simulink model "TRAMI_TM_PNT"  (R2018b)
settings: Solver=ode8  StartTime=0  StopTime=end_time  FixedStep=sampling_time  RelTol=1e-3
PreLoadFcn:
  | TRAMI_TM_PNT_PreLoad;
values from neighbouring files (symbols this model uses):
  sampling_time = 0.0025    [METI_TRAMI_Thermal_ver01_Jmaab_PreLoad.m]
settings Model: Creator=nishimura  LastModifiedBy=E00026
settings DataIOCC: LimitDataPoints=on  SaveFormat=Array  SaveOutput=off  InspectSignalLogs=on  SaveTime=off
settings OptimizationCC: BlockReduction=off  BooleanDataType=off  LifeSpan=inf
settings DebuggingCC: SaveWithParameterizedLinksMsg=none  UnderspecifiedInitializationDetection=Classic  MergeDetectMultiDrivingBlocksExec=none  SignalResolutionControl=TryResolveAllWithWarning  ParameterPrecisionLossMsg=none  StrictBusMsg=ErrorOnBusTreatedAsVector  SFUnexpectedBacktrackingDiag=warning  SFNoUnconditionalDefaultTransitionDiag=warning  SFExecutionAtInitializationDiag=none
settings HardwareCC: ProdBitPerPointer=32  ProdBitPerSizeT=32  ProdBitPerPtrDiffT=32  ProdLargestAtomicFloat=None  ProdIntDivRoundTo=Undefined  ProdEndianess=Unspecified  ProdWordSize=32  ProdHWDeviceType=32-bit Generic  TargetUnknown=on
settings ModelReferenceCC: PropagateSignalLabelsOutOfModel=off
settings SFSimCC: SimUseLocalCustomCode=off
settings RTWCC: RTWUseLocalCustomCode=off
settings CodeAppCC: StateflowObjectComments=on
settings GRTTargetCC: TargetLangStandard=C89/C90 (ANSI)  GeneratePreprocessorConditionals=Disable all
settings ConfigComp: CovMetricSettings=dw  CovHtmlReporting=on  CovSaveCumulativeToWorkspaceVar=on  CovSaveSingleToWorkspaceVar=on  CovExternalEMLEnable=off  CovSFcnEnable=off

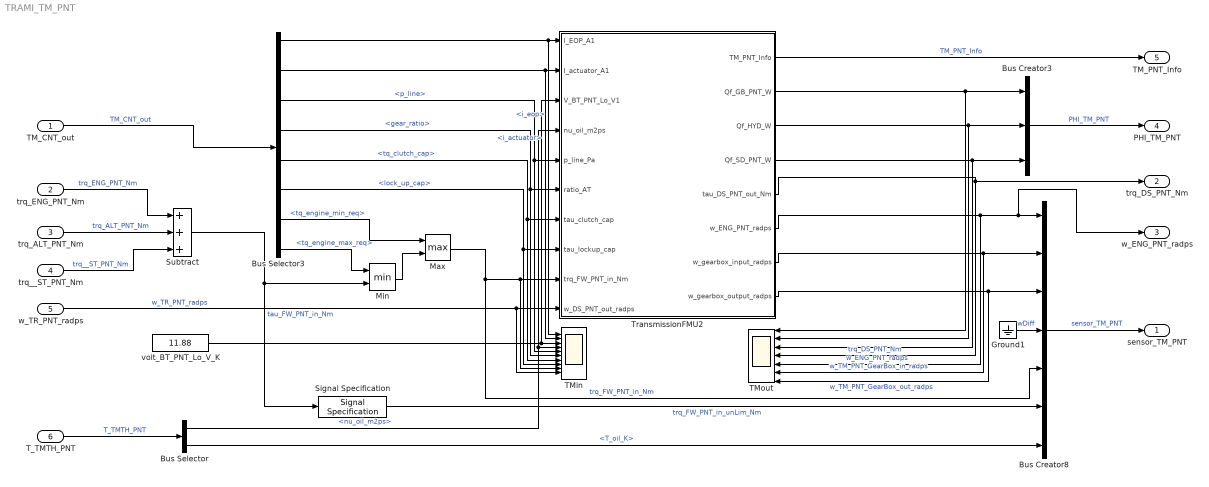
== system TRAMI_TM_PNT ==
  TM_CNT_out : Inport  OutDataTypeStr=Bus: TM_CNT_TRAMI_out  SampleTime=sampling_time
      settings: AttributesFormatString=|
      | <SampleTime = %<SampleTime>>
      | <%<OutDataTypeStr>>
  trq_ENG_PNT_Nm : Inport  Port=2  OutDataTypeStr=double  PortDimensions=1  SampleTime=sampling_time
      settings: AttributesFormatString=<SampleTime = %<SampleTime>>
  trq_ALT_PNT_Nm : Inport  Port=3  OutDataTypeStr=double  PortDimensions=1  SampleTime=sampling_time
      settings: AttributesFormatString=<SampleTime = %<SampleTime>>
  trq__ST_PNT_Nm : Inport  Port=4  OutDataTypeStr=double  PortDimensions=1
      settings: AttributesFormatString=<SampleTime = %<SampleTime>>
  w_TR_PNT_radps : Inport  Port=5  OutDataTypeStr=double  PortDimensions=1
      settings: AttributesFormatString=<SampleTime = %<SampleTime>>
  T_TMTH_PNT : Inport  Port=6  OutDataTypeStr=Bus: T_TMTH_PNT_TRAMI  SampleTime=sampling_time
      settings: AttributesFormatString=|
      | <SampleTime = %<SampleTime>>
      | <%<OutDataTypeStr>>
  Bus Creator3 : BusCreator  Inputs=3
  Bus Creator8 : BusCreator  Inputs=7
  Bus Selector : BusSelector  OutputSignals=nu_oil_m2ps,T_oil_K
  Bus Selector3 : BusSelector  OutputSignals=i_eop,i_actuator,p_line,gear_ratio,tq_clutch_cap,lock_up_cap,tq_engine_min_req,tq_engine_max_req
  Ground1 : Ground
  Max : MinMax  Function=max  Inputs=2
  Min : MinMax  Inputs=2
  Signal Specification : SignalSpecification
  Subtract : Sum  Inputs=3
  TMin : Scope  NumInputPorts=10
  TMout : Scope  NumInputPorts=7
  TransmissionFMU2 : Subsystem
  volt_BT_PNT_Lo_V_K : Constant  Value=11.88
  sensor_TM_PNT : Outport  OutDataTypeStr=Bus: sensor_TM_PNT_TRAMI
      settings: AttributesFormatString=|
      | <SampleTime = %<SampleTime>>
      | <%<OutDataTypeStr>>
  trq_DS_PNT_Nm : Outport  Port=2  OutDataTypeStr=double  PortDimensions=1
      settings: AttributesFormatString=<SampleTime = %<SampleTime>>
  w_ENG_PNT_radps : Outport  Port=3  OutDataTypeStr=double  PortDimensions=1
      settings: AttributesFormatString=<SampleTime = %<SampleTime>>
  PHI_TM_PNT : Outport  Port=4  OutDataTypeStr=Bus: PHI_TM_PNT_TRAMI
      settings: AttributesFormatString=|
      | <SampleTime = %<SampleTime>>
      | <%<OutDataTypeStr>>
  TM_PNT_Info : Outport  Port=5  OutDataTypeStr=Bus: TM_PNT_TRAMI_Info
      settings: AttributesFormatString=|
      | <SampleTime = %<SampleTime>>
      | <%<OutDataTypeStr>>
  wires:
  Min/1 -> Max/2
  Bus Selector3/5 -> TMin/7, TransmissionFMU2/7(tau_clutch_cap)  "<tq_clutch_cap>"
  trq__ST_PNT_Nm/1 -> Subtract/3  "trq__ST_PNT_Nm"
  TM_CNT_out/1 -> Bus Selector3/1  "TM_CNT_out"
  w_TR_PNT_radps/1 -> TMin/10, TransmissionFMU2/10(w_DS_PNT_out_radps)  "w_TR_PNT_radps"
  Bus Selector3/3 -> TMin/5, TransmissionFMU2/5(p_line_Pa)  "<p_line>"
  TransmissionFMU2/5(tau_DS_PNT_out_Nm) -> TMout/4, trq_DS_PNT_Nm/1  "trq_DS_PNT_Nm"
  volt_BT_PNT_Lo_V_K/1 -> TMin/3, TransmissionFMU2/3(V_BT_PNT_Lo_V1)
  Signal Specification/1 -> Bus Creator8/6  "trq_FW_PNT_in_unLim_Nm"
  Subtract/1 -> Signal Specification/1, Min/2  "tau_FW_PNT_in_Nm"
  TransmissionFMU2/6(w_ENG_PNT_radps) -> Bus Creator8/1, w_ENG_PNT_radps/1, TMout/5  "w_ENG_PNT_radps"
  TransmissionFMU2/8(w_gearbox_output_radps) -> Bus Creator8/3, TMout/7  "w_TM_PNT_GearBox_out_radps"
  Max/1 -> TMin/9, TransmissionFMU2/9(trq_FW_PNT_in_Nm), Bus Creator8/5  "trq_FW_PNT_in_Nm"
  Bus Selector/2 -> Bus Creator8/7  "<T_oil_K>"
  TransmissionFMU2/7(w_gearbox_input_radps) -> Bus Creator8/2, TMout/6  "w_TM_PNT_GearBox_in_radps"
  trq_ENG_PNT_Nm/1 -> Subtract/1  "trq_ENG_PNT_Nm"
  Bus Creator3/1 -> PHI_TM_PNT/1  "PHI_TM_PNT"
  Bus Selector3/4 -> TMin/6, TransmissionFMU2/6(ratio_AT)  "<gear_ratio>"
  Bus Selector3/1 -> TransmissionFMU2/1(I_EOP_A1), TMin/1  "<i_eop>"
  TransmissionFMU2/4(Qf_SD_PNT_W) -> Bus Creator3/3, TMout/3
  TransmissionFMU2/1(TM_PNT_Info) -> TM_PNT_Info/1  "TM_PNT_Info"
  TransmissionFMU2/2(Qf_GB_PNT_W) -> Bus Creator3/1, TMout/1
  T_TMTH_PNT/1 -> Bus Selector/1  "T_TMTH_PNT"
  Ground1/1 -> Bus Creator8/4  "wDiff"
  TransmissionFMU2/3(Qf_HYD_W) -> Bus Creator3/2, TMout/2
  Bus Selector3/2 -> TMin/2, TransmissionFMU2/2(I_actuator_A1)  "<i_actuator>"
  Bus Selector3/7 -> Max/1  "<tq_engine_min_req>"
  Bus Selector3/8 -> Min/1  "<tq_engine_max_req>"
  trq_ALT_PNT_Nm/1 -> Subtract/2  "trq_ALT_PNT_Nm"
  Bus Selector/1 -> TMin/4, TransmissionFMU2/4(nu_oil_m2ps)  "<nu_oil_m2ps>"
  Bus Selector3/6 -> TMin/8, TransmissionFMU2/8(tau_lockup_cap)  "<lock_up_cap>"
  Bus Creator8/1 -> sensor_TM_PNT/1  "sensor_TM_PNT"

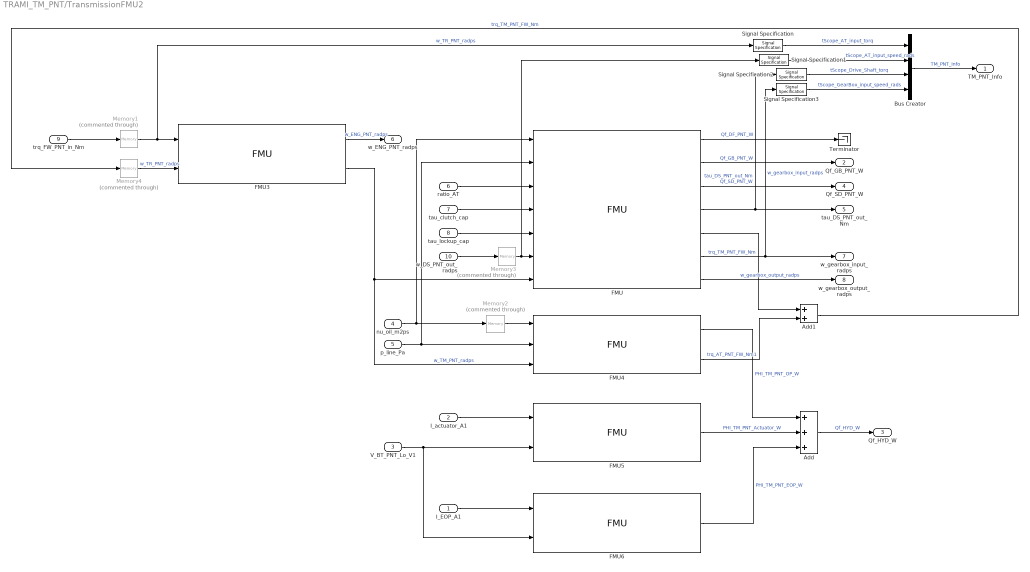
== system TRAMI_TM_PNT/TransmissionFMU2 ==
  I_EOP_A1 : Inport
  I_actuator_A1 : Inport  Port=2
  V_BT_PNT_Lo_V1 : Inport  Port=3
  nu_oil_m2ps : Inport  Port=4
  p_line_Pa : Inport  Port=5
  ratio_AT : Inport  Port=6
  tau_clutch_cap : Inport  Port=7
  tau_lockup_cap : Inport  Port=8
  trq_FW_PNT_in_Nm : Inport  Port=9
  w_DS_PNT_out_radps : Inport  Port=10
  Add : Sum  Inputs=+++
  Add1 : Sum
  Bus Creator : BusCreator  Inputs=4
  FMU : FMU  FMUName=AtDsFmu.fmu  FMUMode=CoSimulation  minsamplestep=2.50000000000000000e-02  binfilename=DISABLED  mask(AtDsFmu [Co-Simulation, v2.0]){}
      mask Display:
      | disp('AtDsFmu');
      | port_label('output',1,'Qf_DF_PNT_W');
      | port_label('output',2,'Qf_GB_PNT_W');
      | port_label('output',3,'Qf_SD_PNT_W');
      | port_label('output',4,'tau_DS_PNT_out_Nm');
      | port_label('output',5,'trq_TM_PNT_FW_Nm');
      | port_label('output',6,'w_gearbox_input_radps');
      | port_label('output',7,'w_gearbox_output_radps');
      | port_label('input',1,'nu_oil_m2ps');
      | port_label('input',2,'p_line_Pa');
      | port_label('input',3,'ratio_AT');
      | port_label('input',4,'tau_clutch_cap');
      | port_label('input',5,'tau_lockup_cap');
      | port_label('input',6,'w_DS_PNT_out_radps');
      | port_label('input',7,'w_TM_PNT_FW_radps');
  FMU3 : FMU  FMUName=Flywheel.fmu  FMUMode=CoSimulation  Iwh=4.00000000000000000e-01  minsamplestep=2.50000000000000000e-02  binfilename=DISABLED  mask(Flywheel [Co-Simulation, v2.0]){}
      mask Display:
      | disp('Flywheel');
      | port_label('output',1,'w_ENG_PNT_radps');
      | port_label('output',2,'w_TM_PNT_FW_radps');
      | port_label('input',1,'trq_ENG_PNT_in_Nm');
      | port_label('input',2,'trq_TM_PNT_FW_Nm');
  FMU4 : FMU  FMUName=OilPump.fmu  FMUMode=CoSimulation  Oil_Viscosity_Breakpoint_2=1.02000000000000000e-05  Oil_Viscosity_Breakpoint_3=1.69000000000000000e-05  Oil_Viscosity_Breakpoint_4=3.12000000000000000e-05  minsamplestep=2.50000000000000000e-02  binfilename=DISABLED  mask(OilPump [Co-Simulation, v2.0]){}
      mask Display:
      | disp('OilPump');
      | port_label('output',1,'PHI_TM_PNT_OP_W');
      | port_label('output',2,'trq_AT_PNT_Nm1');
      | port_label('input',1,'nu_oil_m2ps');
      | port_label('input',2,'p_Line_Pa');
      | port_label('input',3,'w_AT_PNT_radps1');
  FMU5 : FMU  FMUName=ActuatorELoss.fmu  FMUMode=CoSimulation  minsamplestep=2.50000000000000000e-02  binfilename=DISABLED  mask(ActuatorELoss [Co-Simulation, v2.0]){}
      mask Display:
      | disp('ActuatorELoss');
      | port_label('output',1,'PHI_TM_PNT_Actuator_W');
      | port_label('input',1,'I_actuator_A');
      | port_label('input',2,'V_BT_PNT_Lo_V');
  FMU6 : FMU  FMUName=EOPELoss.fmu  FMUMode=CoSimulation  minsamplestep=2.50000000000000000e-02  binfilename=DISABLED  mask(EOPELoss [Co-Simulation, v2.0]){}
      mask Display:
      | disp('EOPELoss');
      | port_label('output',1,'PHI_TM_PNT_EOP_W');
      | port_label('input',1,'I_EOP_A');
      | port_label('input',2,'V_BT_PNT_Lo_V');
  Memory{1..4} (4 alike) : Memory  Commented=through
  Signal Specification{,1..3} (4 alike) : SignalSpecification
  Terminator : Terminator
  TM_PNT_Info : Outport
  Qf_GB_PNT_W : Outport  Port=2
  Qf_HYD_W : Outport  Port=3
  Qf_SD_PNT_W : Outport  Port=4
  tau_DS_PNT_out_Nm : Outport  Port=5
  w_ENG_PNT_radps : Outport  Port=6
  w_gearbox_input_radps : Outport  Port=7
  w_gearbox_output_radps : Outport  Port=8
  wires:
  Signal Specification3/1 -> Bus Creator/4  "tScope_GearBox_input_speed_rads"
  Signal Specification2/1 -> Bus Creator/3  "tScope_Drive_Shaft_torq"
  Signal Specification1/1 -> Bus Creator/2  "tScope_AT_input_speed_rads"
  Signal Specification/1 -> Bus Creator/1  "tScope_AT_input_torq"
  Bus Creator/1 -> TM_PNT_Info/1  "TM_PNT_Info"
  Memory3/1 -> FMU/6, Signal Specification1/1
  Memory4/1 -> FMU3/2  "w_TR_PNT_radps"
  w_DS_PNT_out_radps/1 -> Memory3/1
  Memory1/1 -> FMU3/1, Signal Specification/1  "w_TR_PNT_radps"
  Memory2/1 -> FMU4/1
  FMU/7 -> w_gearbox_output_radps/1  "w_gearbox_output_radps"
  FMU/6 -> Signal Specification3/1, w_gearbox_input_radps/1  "w_gearbox_input_radps"
  FMU/4 -> tau_DS_PNT_out_Nm/1, Signal Specification2/1  "tau_DS_PNT_out_Nm"
  FMU/3 -> Qf_SD_PNT_W/1  "Qf_SD_PNT_W"
  FMU/2 -> Qf_GB_PNT_W/1  "Qf_GB_PNT_W"
  FMU/1 -> Terminator/1  "Qf_DF_PNT_W"
  FMU/5 -> Add1/1  "trq_TM_PNT_FW_Nm"
  tau_lockup_cap/1 -> FMU/5
  tau_clutch_cap/1 -> FMU/4
  ratio_AT/1 -> FMU/3
  Add1/1 -> Memory4/1  "trq_TM_PNT_FW_Nm"
  FMU3/2 -> FMU4/3, FMU/7  "w_TM_PNT_radps"
  nu_oil_m2ps/1 -> Memory2/1, FMU/1
  p_line_Pa/1 -> FMU4/2, FMU/2
  trq_FW_PNT_in_Nm/1 -> Memory1/1
  V_BT_PNT_Lo_V1/1 -> FMU5/2, FMU6/2
  I_actuator_A1/1 -> FMU5/1
  I_EOP_A1/1 -> FMU6/1
  FMU4/2 -> Add1/2  "trq_AT_PNT_FW_Nm1"
  Add/1 -> Qf_HYD_W/1  "Qf_HYD_W"
  FMU4/1 -> Add/1  "PHI_TM_PNT_OP_W"
  FMU6/1 -> Add/3  "PHI_TM_PNT_EOP_W"
  FMU5/1 -> Add/2  "PHI_TM_PNT_Actuator_W"
  FMU3/1 -> w_ENG_PNT_radps/1  "w_ENG_PNT_radps"
